simulink model "Lab08Exp"  (Simulink 7.1)
settings: Solver=ode45  StartTime=0.0  StopTime=10.0  RelTol=1e-3
libraries: simulink x9
settings Model: Creator=George  LastModifiedBy=George

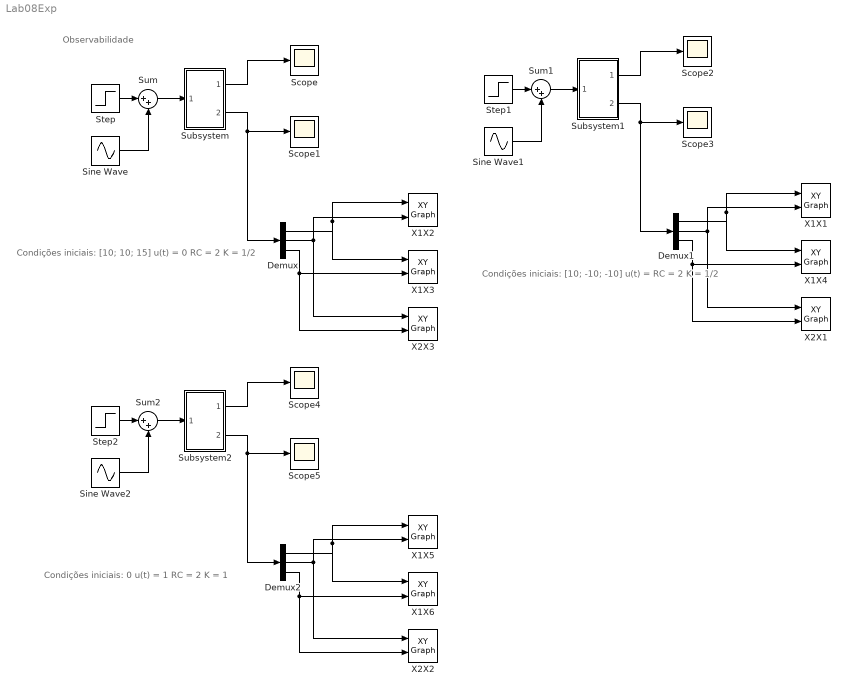
== system Lab08Exp ==
  note: Observabilidade
  note: Condições iniciais:
      | [10; 10; 15]
      | u(t) = 0
      | RC = 2
      | K = 1/2
  note: Condições iniciais:
      | [10; -10; -10]
      | u(t) =
      | RC = 2
      | K = 1/2
  note: Condições iniciais:
      | 0
      | u(t) = 1
      | RC = 2
      | K = 1
  Demux : Demux  Outputs=3
  Demux1 : Demux  Outputs=3
  Demux2 : Demux  Outputs=3
  Scope{,1..5} (6 alike) : Scope
      Scope2 settings: SaveName=ScopeData2
      Scope3 settings: SaveName=ScopeData3
      Scope4 settings: SaveName=ScopeData4
      Scope5 settings: SaveName=ScopeData5
  Sine Wave : Sin  Amplitude=0  Frequency=5  SampleTime=0
  Sine Wave1 : Sin  Amplitude=0  Frequency=5  SampleTime=0
  Sine Wave2 : Sin  Amplitude=0  Frequency=5  SampleTime=0
  Step : Step  Time=0  After=0  SampleTime=0
  Step1 : Step  Time=0  After=0  SampleTime=0
  Step2 : Step  Time=0  SampleTime=0
  Subsystem : Subsystem  mask{RC=2, K=1/2}
  Subsystem1 : Subsystem  mask{RC=2, K=1/2}
  Subsystem2 : Subsystem  mask{RC=2, K=1}
  Sum : Sum  Inputs=|++  OutDataType=sfix(16)  OutScaling=2^0
  Sum1 : Sum  Inputs=|++  OutDataType=sfix(16)  OutScaling=2^0
  Sum2 : Sum  Inputs=|++  OutDataType=sfix(16)  OutScaling=2^0
  X1X{1..6} (6 alike) : simulink/Sinks/XY Graph  SystemSampleTime=-1  xmin=-1  xmax=1  ymin=-1  ymax=1  st=-1
  X2X1 : simulink/Sinks/XY Graph  SystemSampleTime=-1  xmin=-1  xmax=1  ymin=-1  ymax=1  st=-1
  X2X2 : simulink/Sinks/XY Graph  SystemSampleTime=-1  xmin=-1  xmax=1  ymin=-1  ymax=1  st=-1
  X2X3 : simulink/Sinks/XY Graph  SystemSampleTime=-1  xmin=-1  xmax=1  ymin=-1  ymax=1  st=-1
  wires:
  Step/1 -> Sum/1
  Sine Wave/1 -> Sum/2
  Sum/1 -> Subsystem/1(In1)
  Subsystem/1(Out1) -> Scope/1
  Subsystem/2(Out2) -> Scope1/1, Demux/1
  Demux/1 -> X1X2/1, X1X3/1
  Demux/3 -> X1X3/2, X2X3/2
  Demux/2 -> X1X2/2, X2X3/1
  Step1/1 -> Sum1/1
  Sine Wave1/1 -> Sum1/2
  Sum1/1 -> Subsystem1/1(In1)
  Subsystem1/1(Out1) -> Scope2/1
  Subsystem1/2(Out2) -> Scope3/1, Demux1/1
  Demux1/1 -> X1X1/1, X1X4/1
  Demux1/3 -> X1X4/2, X2X1/2
  Demux1/2 -> X1X1/2, X2X1/1
  Step2/1 -> Sum2/1
  Sine Wave2/1 -> Sum2/2
  Sum2/1 -> Subsystem2/1(In1)
  Subsystem2/1(Out1) -> Scope4/1
  Subsystem2/2(Out2) -> Scope5/1, Demux2/1
  Demux2/1 -> X1X5/1, X1X6/1
  Demux2/3 -> X1X6/2, X2X2/2
  Demux2/2 -> X1X5/2, X2X2/1

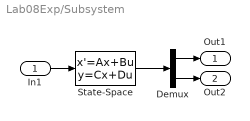
== system Lab08Exp/Subsystem ==
  In1 : Inport
  Demux : Demux  Outputs=[1 3]
  State-Space : StateSpace  A=[(-1/RC)*(2-K) (1/RC)*K -1/RC ; (1/RC)*K (1/RC)*K -1/RC ; (1/(2*RC))*(1+2*K) (1/(2*RC))*(1+2*K) -1/RC]  B=[1/RC*(2-K) ; (-1/RC)*K ; (-1/RC)*K]  C=[-(1+K) -(1+K) 0 ; 1 0 0 ; 0 1 0 ; 0 0 1]  D=[1+K ; 0 ; 0 ; 0]  X0=[10; 10; 15]
  Out1 : Outport
  Out2 : Outport  Port=2
  wires:
  State-Space/1 -> Demux/1
  Demux/1 -> Out1/1
  In1/1 -> State-Space/1
  Demux/2 -> Out2/1

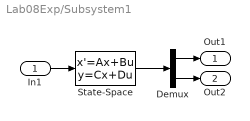
== system Lab08Exp/Subsystem1 ==
  In1 : Inport
  Demux : Demux  Outputs=[1 3]
  State-Space : StateSpace  A=[(-1/RC)*(2-K) (1/RC)*K -1/RC ; (1/RC)*K (1/RC)*K -1/RC ; (1/(2*RC))*(1+2*K) (1/(2*RC))*(1+2*K) -1/RC]  B=[1/RC*(2-K) ; (-1/RC)*K ; (-1/RC)*K]  C=[-(1+K) -(1+K) 0 ; 1 0 0 ; 0 1 0 ; 0 0 1]  D=[1+K ; 0 ; 0 ; 0]  X0=[10; -10; -10]
  Out1 : Outport
  Out2 : Outport  Port=2
  wires:
  State-Space/1 -> Demux/1
  Demux/1 -> Out1/1
  In1/1 -> State-Space/1
  Demux/2 -> Out2/1

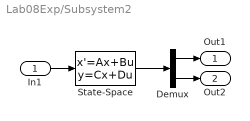
== system Lab08Exp/Subsystem2 ==
  In1 : Inport
  Demux : Demux  Outputs=[1 3]
  State-Space : StateSpace  A=[(-1/RC)*(2-K) (1/RC)*K -1/RC ; (1/RC)*K (1/RC)*K -1/RC ; (1/(2*RC))*(1+2*K) (1/(2*RC))*(1+2*K) -1/RC]  B=[1/RC*(2-K) ; (-1/RC)*K ; (-1/RC)*K]  C=[-(1+K) -(1+K) 0 ; 1 0 0 ; 0 1 0 ; 0 0 1]  D=[1+K ; 0 ; 0 ; 0]
  Out1 : Outport
  Out2 : Outport  Port=2
  wires:
  State-Space/1 -> Demux/1
  Demux/1 -> Out1/1
  In1/1 -> State-Space/1
  Demux/2 -> Out2/1
